simulink model "SimulateHVDC"  (R2024b)
settings: Solver=VariableStepAuto  StartTime=0.0  StopTime=Tf  FixedStep=Ti  MaxStep=Ti  RelTol=1e-6
InitFcn:
  | sim_initHVDC
StartFcn:
  | sim_initHVDC
undefined symbols (not defined in the file): CCMPC, CEMPC, DiscIntNeverNeededParam, GCC, M2C, PCC, plecs, PLL, RFT, TEB, Ti, Ts_cc, Ts_ce, Xmax, Ymax
libraries: slpidlib x5, dspstat3 x5, simulink_extras x2, spsdq0toAlphaBetaZeroLib x2, spsAlphaBetaZerotodq0Lib x2, spsabctoAlphaBetaZeroLib x2, rllib x1, deeplib x1, embmathops x1, spsabctodq0Lib x1, spsAlphaBetaZerotoabcLib x1
(part 2 of 2)

== matlab function SimulateHVDC/Predict basic current and voltages ==
  data: vxy input; VB output; ixy input; wy input; IB output; RFT parameter; M2C parameter; CEMPC parameter
function [VB, IB] = pred(vxy, ixy, wy, RFT, M2C, CEMPC)
%#codegen

% vxy: (p+q) x Np
% ixy: (p+q) x Np
% VB: m x Np
% IB: m x Np

% VB = zeros(m, Np);
% IB = zeros(m, Np);
VB = zeros(6, 1);
IB = zeros(6, 1);

persistent p Np Ts Tab2abc Tabc2ab A pinvA
if isempty(p)
    p       = M2C.p;
    Np      = CEMPC.Np;
    Ts      = CEMPC.Ts;
    Tab2abc = RFT.ab2abc;
    Tabc2ab = RFT.abc2ab;
    A       = M2C.A;
    pinvA   = M2C.pinvA;
end

if Np > 1

    %%% Input port
    VX = repmat(vxy(1:p), 1, Np-1);
    IX = repmat(ixy(1:p), 1, Np-1);

    %%% Output port
    % Rotation matrix
    angles   = (1:Np-1) * (wy * Ts);
    cos_vals = cos(angles);
    sin_vals = sin(angles);
    ROTy     = reshape([cos_vals; -sin_vals; sin_vals; cos_vals], 2, 2*(Np-1))';

    % Predict
    VY = Tab2abc * reshape(ROTy * Tabc2ab * vxy(p+1:end), 2, Np-1);
    IY = Tab2abc * reshape(ROTy * Tabc2ab * ixy(p+1:end), 2, Np-1);

    %%% Predictions formatting
    
    % Concatenate input/output predictions
    VXY = [VX; VY];
    IXY = [IX; IY];
    
    % Add actual measurement as first predicted step
    VXY = [vxy, VXY];
    IXY = [ixy, IXY];
else
    VXY = vxy;
    IXY = ixy;
end

VB(:) = A' * VXY;
IB(:) = pinvA * IXY;
end

== matlab function SimulateHVDC/CMV saturation ==
  data: vo_ref input; Vc input; vo_ref output; vB input
function vo_ref  = vo_sat(vo_ref, Vc, vB)

% The CE MPC operates at slower rate than the LICCs control, hence, if
% the CMV is on the CE MPC limit, the LICCs MPC could result infeasible as
% the external voltages keep changing after the CE MPC computation.
% This saturation operates at the LICCs MPC rate.

vo_max = min([Vc(1:3); zeros(3, 1)] - vB);
vo_min = max([zeros(3, 1); -Vc(4:6)] - vB);
vo_ref = max([min([vo_ref, vo_max])], vo_min);

== matlab function SimulateHVDC/Subsystem/MATLAB Function ==
  data: Vc input; vo_max output; vB input; vo_min output
function [vo_max, vo_min] = vo_lim(Vc, vB)

vo_max = min([Vc(1:3); zeros(3, 1)] - vB);
vo_min = max([zeros(3, 1); -Vc(4:6)] - vB);

== matlab function SimulateHVDC/NN CEC/Input format ==
  data: Ec input; iP input; im_ab input; vm_ab input; wy input; ie_mpc input; vo_mpc input; obs output; M2C parameter; RFT parameter; Xmax parameter
function obs = input(Ec, iP, im_ab, vm_ab, wy, ie_mpc, vo_mpc, M2C, RFT, Xmax)
%#codegen

persistent Ec_ref Tab2abc
if isempty(Ec_ref)
    Ec_ref = M2C.Ec_ref;
    Tab2abc = RFT.ab2abc;
end

% Machine alpha-beta variables
pm = 3/2 * (vm_ab(1) * im_ab(1) + vm_ab(2) * im_ab(2));
qm = 3/2 * (vm_ab(2) * im_ab(1) - vm_ab(1) * im_ab(2));
sm = [pm; qm];

% % Machine line variables
% im_abc = Tab2abc * im_ab;
% vm_abc = Tab2abc * vm_ab;
% p1  = (vm_abc(1) - vm_abc(3)) * im_abc(1);
% p2  = (vm_abc(2) - vm_abc(3)) * im_abc(2);
% p12 = [p1; p2];

% Observation
obs = zeros(17, 1);

% FIXED variables
obs(1:6)   = Ec - mean(Ec);
obs(7)     = iP;

% MACHINE alpha-beta variables
obs(8:9)   = im_ab;
obs(10:11) = vm_ab;
obs(12:13) = sm;

% % MACHINE line variables
% obs(8:9)   = im_abc(1:2);
% obs(10:11) = vm_abc(1:2) - vm_abc(3);
% obs(12:13) = p12;

% OPTIONAL
obs(14)    = wy;

% Additional variables
obs(15:16) = ie_mpc;
obs(17)    = vo_mpc;

% Normalize
obs = obs ./ Xmax;

== matlab function SimulateHVDC/Energy balance ==
  data: Ec input; ie_ref output; Vc input; VB input; IB input; vo_ref output; flag output; J output; Nac output; Tex output; M2C parameter; CEMPC parameter
function [ie_ref, vo_ref, flag, J, Nac, Tex] = EMPC(Ec, Vc, VB, IB, M2C, CEMPC)
%#codegen

persistent Ts m n Np K MI NN ONE Nl is_max is_max2 vo_max2 Vc_ref2 Ec_ref Ec_ref2 Hu_z Aineq_z lambda_z Hu_o Aineq_o lambda_o iA_z iA_o options_z options_o Ec_dev
if isempty(Ts)
    Ts       = CEMPC.Ts;
    m        = M2C.m;
    n        = M2C.n;
    Np       = CEMPC.Np;
    K        = CEMPC.K;
    MI       = CEMPC.MI;
    NN       = CEMPC.NN;
    ONE      = CEMPC.ONE;
    Nl       = CEMPC.Nl;
    is_max   = M2C.is_max;
    is_max2  = is_max^2;
    vo_max2  = M2C.vo_max^2;
    Vc_ref2  = M2C.Vc_ref^2;
    Ec_ref   = M2C.Ec_ref;
    Ec_ref2  = Ec_ref^2;
    Hu_z     = CEMPC.Hu_z;
    Aineq_z  = CEMPC.Aineq_z;
    lambda_z = CEMPC.lambda_z;
    Hu_o     = CEMPC.Hu_o;
    Aineq_o  = CEMPC.Aineq_o;
    lambda_o = CEMPC.lambda_o;
    Ec_dev   = M2C.Ec_dev;
    iA_z     = false(size(zeros(2 * m * Np, 1)));
    iA_o     = false(size(zeros(2 * Np, 1)));
    options_z                     = mpcActiveSetOptions;
    options_z.MaxIterations       = 20;
    options_z.ConstraintTolerance = 1e-4;
    options_o                     = mpcActiveSetOptions;
    options_o.MaxIterations       = 10;
    options_o.ConstraintTolerance = 1e-4;
end

tic

% Preallocation
vo_ref_temp = zeros(Np, 1);
ie_ref_temp = zeros(n*Np, 1);
flag_z = int32(0);
flag_o = int32(0);
vs_temp = zeros(m*Np, 1);
is_temp = zeros(m*Np, 1);

for l = 1:Nl
    %%% LICCs subproblem Jz = Jz_x + Jz_u

    % Initialization
    % vs_temp(:) = VB(:) + ONE * vo_ref_temp;
    vs_temp = VB + vo_ref_temp';
    vs_temp = vs_temp(:);

    % Linear model matrices
    E = Ts * K * diag(vs_temp); % Disturbances matrix
    B = E * NN;                 % Input matrix
    P = IB(:);                  % Disturbances

    % State reference tracking Jx_z, quadratic and linear terms 
    Hx_z = 2 * B' * MI * B / (Ec_ref2*Ec_dev^2);
    fx_z = 2 * B' * MI * (repmat(Ec, Np, 1) + E * P) / (Ec_ref2*Ec_dev^2);

    % Control action penalization Ju_z, linear term
    fu_z = 2 * NN' * IB(:) / is_max2;

    % Total cost function J_z
    H_z = Hx_z + lambda_z * Hu_z;
    f_z = fx_z + lambda_z * fu_z;
    
    % Constraints
    ub      =  is_max - IB(:);
    lb      = -is_max - IB(:);
    bineq_z = [ub; -lb];

    % Solve
    [ie_ref_temp, flag_z, iA_z] = mpcActiveSetSolver(H_z, f_z, Aineq_z, bineq_z, zeros(0, n*Np), zeros(0, 1), iA_z, options_z);

    %%% CMV subproblem Jo = Jo_x + Jo_u

    % Initialization
    is_temp = IB(:) + NN * ie_ref_temp;

    % Linear model matrices
    E = Ts * K * diag(is_temp); % Distrubances matrix
    B = E * ONE;                % Input matrix
    P = VB(:);                  % Distrubances

    % State reference tracking Jx_o, quadratic and linear terms 
    Hx_o = 2 * B' * MI * B / (Ec_ref2*Ec_dev^2);
    fx_o = 2 * B' * MI * (repmat(Ec, Np, 1) + E * P) / (Ec_ref2*Ec_dev^2);

    % Control action penalization Jo_u
    fu_o = zeros(Np, 1) / vo_max2;

    % Total cost function J_o
    H_o = Hx_o + lambda_o * Hu_o;
    f_o = fx_o + lambda_o * fu_o;

    % Constraints
    ub = min([Vc(1:3); 0; 0; 0] - VB, [], 1)';
    lb = max([0; 0; 0; -Vc(4:6)] - VB, [], 1)';
    bineq_o = [ub; -lb];

    % Solve
    [vo_ref_temp, flag_o, iA_o] = mpcActiveSetSolver(H_o, f_o, Aineq_o, bineq_o, zeros(0, Np), zeros(0, 1), iA_o, options_o);
end

% ie_ref = ie_ref_temp(1:n);
ie_ref = ie_ref_temp(1:2);
vo_ref = vo_ref_temp(1);

if and(0 < flag_z, 0 < flag_o)
    flag_T = 1;
else
    flag_T = -3;
end

vs_temp = VB(:) + ONE * vo_ref_temp;
Ec_pred = Ec + Ts * reshape(vs_temp .* is_temp, m, Np);
Ec_pred = Ec_pred(:);
J_E = sum((Ec_pred - mean(Ec_pred)).^2) / (Ec_ref2*Ec_dev^2);
J_i = sum(is_temp.^2) / is_max2;
J_v = sum(vo_ref_temp.^2) / vo_max2;
J_T = J_E + lambda_z * J_i + lambda_o * J_v;

% flag = [flag_z, flag_o, flag_T];
flag = flag_T;
J = [J_E, J_i, J_v, J_T];
Nac = [sum(iA_z), sum(iA_o)];

Tex = toc;
end

== matlab function SimulateHVDC/Modulation index ==
  data: vs input; D output; Vc input
function D = delta(vs, Vc)
%#codegen

vs(4:6) = -vs(4:6);

% Cluster modulation index
D = zeros(6, 1);
D(:) = min(max(vs ./ Vc, 0), 1);
end

== matlab function SimulateHVDC/NN CEC/Output format ==
  data: act input; iB input; ie output; vo output; Vc input; vB input; Ymax parameter; M2C parameter
function [ie, vo] = output(act, iB, Vc, vB, Ymax, M2C)
%#codegen

persistent is_max Ac  MaxIter lambda Tol n2 Nc
if isempty(Ac)
    is_max  = M2C.is_max;
    Ac      = [M2C.N; -M2C.N];
    MaxIter = 100;
    lambda  = 1;
    Tol     = 1e-3;
    n2      = sum(Ac.^2, 2);
    Nc      = size(Ac, 1);
end

act = act .* Ymax;
ie = act(1:2);
vo = act(3);

% % Clip CMV
% ub = min([Vc(1:3); 0; 0; 0] - vB, [], 1)';
% lb = max([0; 0; 0; -Vc(4:6)] - vB, [], 1)';
% vo = min(max(vo, lb), ub);
% 
% % Project LICCs
% % Initialize projection
% x_proj = ie;
% bc = [is_max - iB; is_max + iB];
% 
% p = zeros(size(Ac));
% for k = 1:MaxIter
%     for i = 1:Nc
%         ai      = Ac(i, :)';
%         bi      = bc(i);
%         aux     = x_proj + p(i, :)';
%         ri      = ai' * aux - bi;
%         delta   = lambda * (ri / n2(i)) * ai * (ri > 0);
%         x_proj  = aux - delta;
%         p(i, :) = delta';
%     end
% 
%     % Max constraint violation
%     error = max(Ac * x_proj - bc);
%     if error < Tol, break; end
% end
% 
% ie = x_proj;

== matlab function SimulateHVDC/LICCs control ==
  data: vse output; ie_ref input; ie input; vsP input; vsm input; vo_ref input; Vc input; flag output; J output; Nac output; Tex output; CCMPC parameter; M2C parameter
function [vse, flag, J, Nac, Tex] = CMPC(ie_ref, ie, vsP, vsm, vo_ref, Vc, CCMPC, M2C)
%#codegen

persistent nu Ad Bd Hx Hu H lambda Aineq is_max is_max2 pinvT vse_prev iA options
if isempty(nu)
    nu       = CCMPC.nu;     % # of control actions
    Ad       = CCMPC.Ad;     % State matrix
    Bd       = CCMPC.Bd;     % Input matrix
    Hx       = CCMPC.Hx;     % Reference tracking Hessian
    Hu       = CCMPC.Hu;     % Control effort Hessian
    H        = CCMPC.H;      % Total control Hessian
    lambda   = CCMPC.lambda; % Control effort weighting factor
    Aineq    = CCMPC.Aineq;  % Control actions constraints matrix
    is_max   = M2C.is_max;   % Max. cluster current
    is_max2  = is_max^2;
    pinvT    = CCMPC.pinvT;
    vse_prev = [0; 0];
    % mpcActiveSetSolver initialization
    iA        = false(size(Aineq, 1), 1);  % Active constraints
    options   = mpcActiveSetOptions;
    options.MaxIterations       = 10;
    options.ConstraintTolerance = 1.0e-5;
end

tic

% Sampling delay compensation
ie = Ad(1:2, 1:2) * ie + Bd(1:2, 1:2) * vse_prev;

% 2-step horizon LICCs references
ie_ref = repmat(ie_ref, 2, 1);

% Reference tracking linear term, normalized (f=fx+fu, fu=0)
f = 2 * Bd' * (-ie_ref + Ad * ie) / is_max2;

% Control action constraints
p  = vo_ref + pinvT(:, 1:3) * [vsP; vsm];
ub = repmat([Vc(1:3); 0; 0; 0] - p, 2, 1);
lb = repmat([0; 0; 0; -Vc(4:6)] - p, 2, 1);
bineq = [ub; -lb];

% Solve
[vse_temp, flag, iA, ~] = mpcActiveSetSolver(H, f, Aineq, bineq, zeros(0, 2*nu), zeros(0, 1), iA, options);
vse = zeros(2, 1);
vse(:) = vse_temp(1:2);

% if flag < 0
%     vse = [0; 0];
% end

% Control summary
Tex = toc;
Nac = sum(iA);
Jx = vse_temp' * Hx * vse_temp + f' * vse_temp;
Ju = vse_temp' * Hu * vse_temp;
JT  =  Jx + lambda * Ju;
J = [Jx, Ju, JT];

vse_prev = vse;
end
